simulink model "c28069_PMDC_PIL"  (R2018b)
settings: Solver=ode4  StartTime=0.0  StopTime=0.12  FixedStep=Tsim  RelTol=1e-3
values from neighbouring files (symbols this model uses):
  B = 1.8026e-4    (= 0.00018026)    [data_init_DC.m]
  imax = 5    [data_init_DC.m]
  J = 3.559e-6    (= 3.559e-06)    [data_init_DC.m]
  kiI = wcI*Ra    (= 3234.89428601)    [data_init_DC.m]
  kiW = wcW*B    (= 0.110231010207)    [data_init_DC.m]
  kpI = wcI*La    (= 5.29)    [data_init_DC.m]
  kpW = wcW*J    (= 0.00217636838637)    [data_init_DC.m]
  Kt = 0.0232    [data_init_DC.m]
  La = 8.6507e-4    (= 0.00086507)    [data_init_DC.m]
  Ra = 0.5290    (= 0.529)    [data_init_DC.m]
  Ts = Tsw    (= 5e-05)    [data_init_DC.m]
  Vdc = 10    [data_init_DC.m]
libraries: simulink x2
settings Model: ExtModeTrigDuration=8  Creator=matti  LastModifiedBy=matti
settings OptimizationCC: DefaultUnderspecifiedDataType=single  MaxStackSize=512
settings DebuggingCC: ParameterTunabilityLossMsg=error
settings HardwareCC: ProdBitPerChar=16  ProdBitPerInt=16  ProdBitPerPointer=32  ProdBitPerSizeT=32  ProdBitPerPtrDiffT=32  ProdLargestAtomicInteger=Integer  ProdLargestAtomicFloat=None  ProdWordSize=16  ProdLongLongMode=on  ProdHWDeviceType=Texas Instruments->C2000
settings SFSimCC: SimUseLocalCustomCode=off  MATLABDynamicMemAlloc=off
settings RTWCC: SystemTargetFile=ert.tlc  HardwareBoard=TI Piccolo F28069M LaunchPad  TemplateMakefile=ert_default_tmf  GenerateReport=on  RTWUseLocalCustomCode=off  Toolchain=Texas Instruments Code Composer Studio (C2000)  IncludeHyperlinkInReport=on  LaunchReport=on  CreateSILPILBlock=PIL  GenerateTraceInfo=on  GenerateTraceReport=on  GenerateTraceReportSl=on  GenerateTraceReportSf=on  GenerateTraceReportEml=on
settings CodeAppCC: ForceParamTrailComments=on  IgnoreCustomStorageClasses=off  OperatorAnnotations=on  SimulinkDataObjDesc=on  SFDataObjDesc=on  MATLABFcnDesc=on  InsertBlockDesc=on  StateflowObjectComments=on  MATLABSourceComments=on
settings ERTTargetCC: CodeReplacementLibrary=TI C28x  MultiwordLength=2048

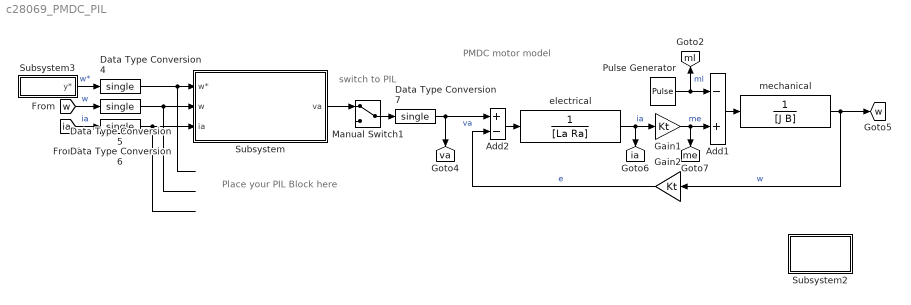
== system c28069_PMDC_PIL ==
  note: PMDC motor model
  note: switch to PIL
  note: Place your PIL Block here
  Add1 : Sum  Inputs=-+
  Add2 : Sum  Inputs=+-
  Data Type Conversion{4..7} (4 alike) : DataTypeConversion  OutDataTypeStr=single
  Gain1 : Gain  Gain=Kt
  Gain2 : Gain  Gain=Kt
  Manual Switch1 : ManualSwitch
  Pulse Generator : DiscretePulseGenerator  PulseType=Time based  Amplitude=0.025  Period=1  PulseWidth=50  PhaseDelay=0.04
  Subsystem : Subsystem
      mask Display: disp('cascade\nspeed/current loops')
  Subsystem2 : Subsystem
      mask Display: disp('stream')
  Subsystem3 : Subsystem
      mask Display: disp('reference')
  electrical : TransferFcn  Denominator=[La Ra]
  mechanical : TransferFcn  Denominator=[J B]
  tag scope: ia=global, me=global, ml=global, va=global, w=global
  wires:
  Add2/1 -> electrical/1
  Add1/1 -> mechanical/1
  Gain1/1 -> Add1/2, [me]  "me"
  electrical/1 -> Gain1/1, [ia]  "ia"
  mechanical/1 -> Gain2/1, [w]  "w"
  Gain2/1 -> Add2/2  "e"
  Pulse Generator/1 -> [ml], Add1/1  "ml"
  Data Type Conversion7/1 -> Add2/1, [va]  "va"
  Subsystem3/1(y*) -> Data Type Conversion4/1  "w*"
  Data Type Conversion4/1 -> Subsystem/1(w*)
  Data Type Conversion5/1 -> Subsystem/2(w)
  [w] -> Data Type Conversion5/1  "w"
  [ia] -> Data Type Conversion6/1  "ia"
  Data Type Conversion6/1 -> Subsystem/3(ia)
  Manual Switch1/1 -> Data Type Conversion7/1
  Subsystem/1(va) -> Manual Switch1/1
  ? -> Manual Switch1/2

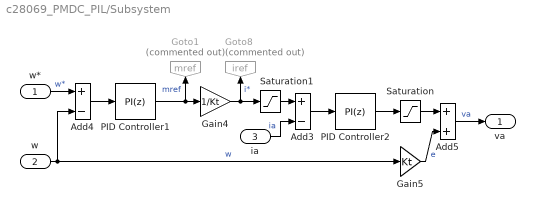
== system c28069_PMDC_PIL/Subsystem ==
  w* : Inport
  w : Inport  Port=2
  ia : Inport  Port=3
  Add3 : Sum  Inputs=+-
  Add4 : Sum  Inputs=+-
  Add5 : Sum
  Gain4 : Gain  Gain=1/Kt
  Gain5 : Gain  Gain=Kt
  Goto1 : Goto  Commented=on  GotoTag=mref  TagVisibility=global
  Goto8 : Goto  Commented=on  GotoTag=iref  TagVisibility=global
  PID Controller1 : simulink/Continuous/PID Controller  Controller=PI  Form=Parallel  TimeDomain=Discrete-time  SampleTime=Ts  IntegratorMethod=Forward Euler  FilterMethod=Forward Euler  ControllerParametersSource=internal  P=kpW  I=kiW  D=0  UseFilter=on  N=100  TunerSelectOption=Transfer Function Based (PID Tuner App)  InitialConditionSource=internal  InitialConditionForIntegrator=0  InitialConditionForFilter=0  DifferentiatorICPrevScaledInput=0  ExternalReset=none  TrackingMode=off  Kt=1  LimitOutput=on  UpperSaturationLimit=Kt*imax  LowerSaturationLimit=-Kt*imax  LinearizeAsGain=on  AntiWindupMode=back-calculation  Kb=kiW/kpW  POutMin=[]  POutMax=[]  IOutMin=[]  IOutMax=[]  DOutMin=[]  DOutMax=[]  NOutMin=[]  NOutMax=[]  SumOutMin=[]  SumOutMax=[]  SaturationOutMin=[]  SaturationOutMax=[]  PParamMin=[]  PParamMax=[]  IParamMin=[]  IParamMax=[]  DParamMin=[]  DParamMax=[]  NParamMin=[]  NParamMax=[]  KbParamMin=[]  KbParamMax=[]  KtParamMin=[]  KtParamMax=[]  KbOutMin=[]  KbOutMax=[]  KtOutMin=[]  KtOutMax=[]  IntegratorOutMin=[]  IntegratorOutMax=[]  FilterOutMin=[]  FilterOutMax=[]  SumI1OutMin=[]  SumI1OutMax=[]  SumI2OutMin=[]  SumI2OutMax=[]  SumI3OutMin=[]  SumI3OutMax=[]  SumI4OutMin=[]  SumI4OutMax=[]  SumDOutMin=[]  SumDOutMax=[]  DifferentiatorOutMin=[]  DifferentiatorOutMax=[]  FilterDiffOutCoefMin=[]  FilterDiffOutCoefMax=[]  ReciprocalOutMin=[]  ReciprocalOutMax=[]  SumDenOutMin=[]  SumDenOutMax=[]  SumNumOutMin=[]  SumNumOutMax=[]  DivideOutMin=[]  DivideOutMax=[]  IntegratorContinuousStateAttributes=''  IntegratorStateMustResolveToSignalObject=off  IntegratorRTWStateStorageClass=Auto  FilterContinuousStateAttributes=''  FilterStateMustResolveToSignalObject=off  FilterRTWStateStorageClass=Auto  ParallelPVariant=InternalParameters  IdealPVariant=Disabled  IVariant=InternalParameters  DVariant=Disabled  IntegratorVariant=Discrete  SatVariant=Enabled  AWVariant=BackCalculation  PCopyVariant=Disabled  TRVariant=Disabled  FdbkBlocksVariant=Forward  IdealPFdbkVariant=Disabled  SatFdbkVariant=Disabled  DerivativeFilterVariant=Disabled  NVariant=Disabled  NCopyVariant=Disabled_SignalSpec  FilterICVariant=Disabled  IntegratorICVariant=InternalICs  ExternalResetVariant=Disabled  TRSumVariant=Passthrough  SumFdbkVariant=Disabled  SumVariant=Sum_PI
  PID Controller2 : simulink/Continuous/PID Controller  Controller=PI  Form=Parallel  TimeDomain=Discrete-time  SampleTime=Ts  IntegratorMethod=Forward Euler  FilterMethod=Forward Euler  ControllerParametersSource=internal  P=kpI  I=kiI  D=0  UseFilter=on  N=100  TunerSelectOption=Transfer Function Based (PID Tuner App)  InitialConditionSource=internal  InitialConditionForIntegrator=0  InitialConditionForFilter=0  DifferentiatorICPrevScaledInput=0  ExternalReset=none  TrackingMode=off  Kt=1  LimitOutput=on  UpperSaturationLimit=Vdc  LowerSaturationLimit=0  LinearizeAsGain=on  AntiWindupMode=back-calculation  Kb=kiI/kpI  POutMin=[]  POutMax=[]  IOutMin=[]  IOutMax=[]  DOutMin=[]  DOutMax=[]  NOutMin=[]  NOutMax=[]  SumOutMin=[]  SumOutMax=[]  SaturationOutMin=[]  SaturationOutMax=[]  PParamMin=[]  PParamMax=[]  IParamMin=[]  IParamMax=[]  DParamMin=[]  DParamMax=[]  NParamMin=[]  NParamMax=[]  KbParamMin=[]  KbParamMax=[]  KtParamMin=[]  KtParamMax=[]  KbOutMin=[]  KbOutMax=[]  KtOutMin=[]  KtOutMax=[]  IntegratorOutMin=[]  IntegratorOutMax=[]  FilterOutMin=[]  FilterOutMax=[]  SumI1OutMin=[]  SumI1OutMax=[]  SumI2OutMin=[]  SumI2OutMax=[]  SumI3OutMin=[]  SumI3OutMax=[]  SumI4OutMin=[]  SumI4OutMax=[]  SumDOutMin=[]  SumDOutMax=[]  DifferentiatorOutMin=[]  DifferentiatorOutMax=[]  FilterDiffOutCoefMin=[]  FilterDiffOutCoefMax=[]  ReciprocalOutMin=[]  ReciprocalOutMax=[]  SumDenOutMin=[]  SumDenOutMax=[]  SumNumOutMin=[]  SumNumOutMax=[]  DivideOutMin=[]  DivideOutMax=[]  IntegratorContinuousStateAttributes=''  IntegratorStateMustResolveToSignalObject=off  IntegratorRTWStateStorageClass=Auto  FilterContinuousStateAttributes=''  FilterStateMustResolveToSignalObject=off  FilterRTWStateStorageClass=Auto  ParallelPVariant=InternalParameters  IdealPVariant=Disabled  IVariant=InternalParameters  DVariant=Disabled  IntegratorVariant=Discrete  SatVariant=Enabled  AWVariant=BackCalculation  PCopyVariant=Disabled  TRVariant=Disabled  FdbkBlocksVariant=Forward  IdealPFdbkVariant=Disabled  SatFdbkVariant=Disabled  DerivativeFilterVariant=Disabled  NVariant=Disabled  NCopyVariant=Disabled_SignalSpec  FilterICVariant=Disabled  IntegratorICVariant=InternalICs  ExternalResetVariant=Disabled  TRSumVariant=Passthrough  SumFdbkVariant=Disabled  SumVariant=Sum_PI
  Saturation : Saturate  UpperLimit=Vdc  LowerLimit=0
  Saturation1 : Saturate  UpperLimit=imax  LowerLimit=-imax
  va : Outport
  wires:
  PID Controller1/1 -> Goto1/1, Gain4/1  "mref"
  Saturation1/1 -> Add3/1
  Gain4/1 -> Goto8/1, Saturation1/1  "i*"
  Add4/1 -> PID Controller1/1
  w/1 -> Add4/2, Gain5/1  "w"
  Add5/1 -> va/1  "va"
  Saturation/1 -> Add5/1
  PID Controller2/1 -> Saturation/1
  Add3/1 -> PID Controller2/1
  Gain5/1 -> Add5/2  "e"
  w*/1 -> Add4/1  "w*"
  ia/1 -> Add3/2  "ia"

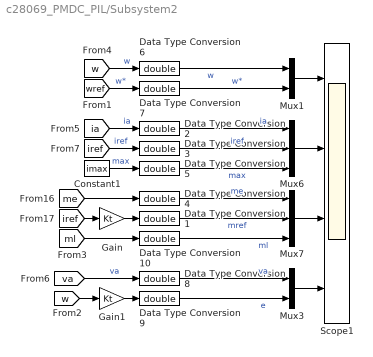
== system c28069_PMDC_PIL/Subsystem2 ==
  Constant1 : Constant  Value=imax  SampleTime=Ts
  Data Type Conversion{1..10} (10 alike) : DataTypeConversion  OutDataTypeStr=double
  Gain : Gain  Gain=Kt
  Gain1 : Gain  Gain=Kt
  Mux1 : Mux  Inputs=2
  Mux3 : Mux  Inputs=2
  Mux6 : Mux  Inputs=3
  Mux7 : Mux  Inputs=3
  Scope1 : Scope  NumInputPorts=4
  wires:
  Mux3/1 -> Scope1/4
  Data Type Conversion8/1 -> Mux3/1  "va"
  [iref] -> Gain/1
  [me] -> Data Type Conversion4/1
  Data Type Conversion5/1 -> Mux6/3  "max"
  Data Type Conversion7/1 -> Mux1/2  "w*"
  Mux1/1 -> Scope1/1
  Data Type Conversion6/1 -> Mux1/1  "w"
  Data Type Conversion2/1 -> Mux6/1  "ia"
  Mux7/1 -> Scope1/3
  Gain/1 -> Data Type Conversion1/1
  Data Type Conversion4/1 -> Mux7/1  "me"
  Data Type Conversion1/1 -> Mux7/2  "mref"
  Data Type Conversion3/1 -> Mux6/2  "iref"
  [ia] -> Data Type Conversion2/1  "ia"
  [iref] -> Data Type Conversion3/1  "iref"
  Constant1/1 -> Data Type Conversion5/1  "max"
  [wref] -> Data Type Conversion7/1  "w*"
  [w] -> Data Type Conversion6/1  "w"
  Mux6/1 -> Scope1/2
  [va] -> Data Type Conversion8/1  "va"
  Data Type Conversion9/1 -> Mux3/2  "e"
  [w] -> Gain1/1
  Gain1/1 -> Data Type Conversion9/1
  [ml] -> Data Type Conversion10/1
  Data Type Conversion10/1 -> Mux7/3  "ml"

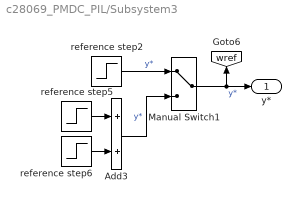
== system c28069_PMDC_PIL/Subsystem3 ==
  Add3 : Sum
  Manual Switch1 : ManualSwitch
  reference step2 : Step  Time=0.01  After=50  SampleTime=Ts
  reference step5 : Step  Time=0.01  After=50  SampleTime=Ts
  reference step6 : Step  Time=0.07  After=-50  SampleTime=Ts
  y* : Outport
  tag scope: wref=global
  wires:
  Manual Switch1/1 -> [wref], y*/1  "y*"
  reference step2/1 -> Manual Switch1/1  "y*"
  reference step6/1 -> Add3/2
  reference step5/1 -> Add3/1
  Add3/1 -> Manual Switch1/2  "y*"
